simulink model "admittance_controller_full"  (R2021b)
settings: Solver=VariableStepAuto  StartTime=0.0  StopTime=25  RelTol=1e-3
settings Model: Creator=Martin  LastModifiedBy=Martin

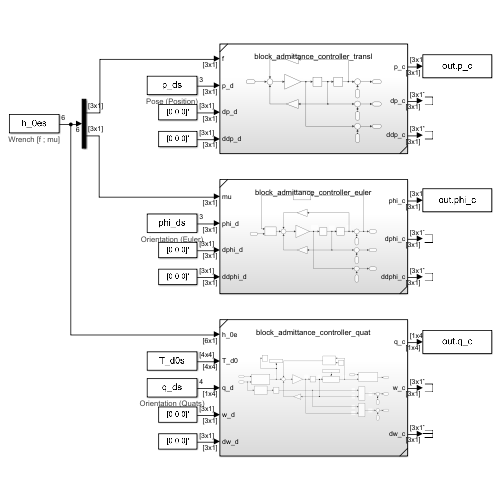
[thumbnail: Simulink's stored preview of the top-level diagram]
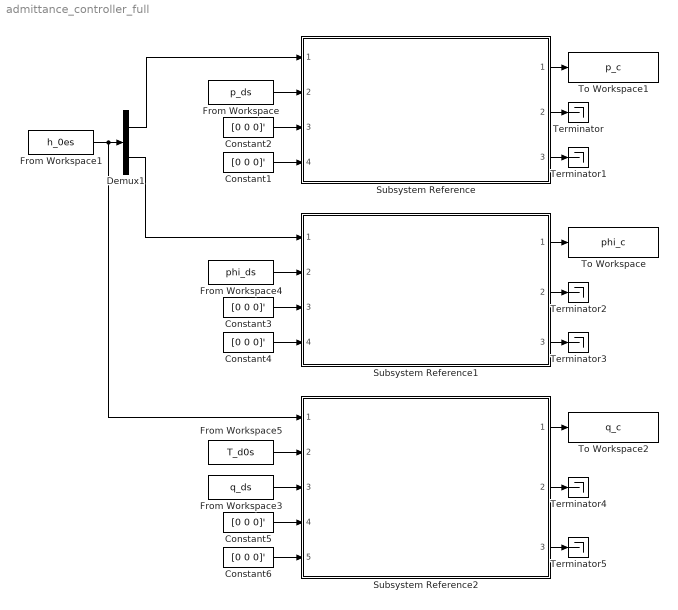
== system admittance_controller_full ==
  Constant{1..6} (6 alike) : Constant  Value=[0 0 0]'  VectorParams1D=off
  Demux1 : Demux  Outputs=2
  From Workspace : FromWorkspace  VariableName=p_ds
      settings: AttributesFormatString=Pose (Position)
  From Workspace1 : FromWorkspace  VariableName=h_0es
      settings: AttributesFormatString=Wrench [f ; mu]
  From Workspace3 : FromWorkspace  VariableName=q_ds
      settings: AttributesFormatString=Orientation (Quats)
  From Workspace4 : FromWorkspace  VariableName=phi_ds
      settings: AttributesFormatString=Orientation (Euler)
  From Workspace5 : FromWorkspace  VariableName=T_d0s
  Subsystem Reference : Subsystem  ReferencedSubsystem=block_admittance_controller_transl
  Subsystem Reference1 : Subsystem  ReferencedSubsystem=block_admittance_controller_euler
  Subsystem Reference2 : Subsystem  ReferencedSubsystem=block_admittance_controller_quat
  Terminator{,1..5} (6 alike) : Terminator
  To Workspace : ToWorkspace  VariableName=phi_c  SampleTime=-1
  To Workspace1 : ToWorkspace  VariableName=p_c  SampleTime=-1
  To Workspace2 : ToWorkspace  VariableName=q_c  SampleTime=-1
  wires:
  Constant1/1 -> Subsystem Reference/4
  From Workspace1/1 -> Subsystem Reference2/1, Demux1/1
  Constant2/1 -> Subsystem Reference/3
  From Workspace3/1 -> Subsystem Reference2/3
  Demux1/2 -> Subsystem Reference1/1
  Demux1/1 -> Subsystem Reference/1
  From Workspace/1 -> Subsystem Reference/2
  Subsystem Reference1/1 -> To Workspace/1
  Subsystem Reference/1 -> To Workspace1/1
  Subsystem Reference2/1 -> To Workspace2/1
  From Workspace4/1 -> Subsystem Reference1/2
  Constant3/1 -> Subsystem Reference1/3
  Constant4/1 -> Subsystem Reference1/4
  Constant5/1 -> Subsystem Reference2/4
  Constant6/1 -> Subsystem Reference2/5
  Subsystem Reference/2 -> Terminator/1
  Subsystem Reference1/2 -> Terminator2/1
  Subsystem Reference2/2 -> Terminator4/1
  Subsystem Reference2/3 -> Terminator5/1
  Subsystem Reference/3 -> Terminator1/1
  Subsystem Reference1/3 -> Terminator3/1
  From Workspace5/1 -> Subsystem Reference2/2
